simulink library "threeSurfaceThreeTether_cl"  (R2018b)
settings: Solver=VariableStepAuto  StartTime=0.0  StopTime=10.0  RelTol=1e-3
libraries: vrlib x4, turbine_ul x2, apparentWind_ul x1, eulAng2RotMat_ul x1, vectorNormalizer_ul x1, avlAerodynamics x1, sixDoFDynamics_ul x1
settings Model: Creator=mcobb  LastModifiedBy=mcobb

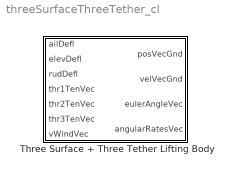
== system threeSurfaceThreeTether_cl ==
  Three Surface + Three Tether Lifting Body : Subsystem  mask{rho=1.225, vol=1, grav=9.81, thr1PosVec=[1 0 0], thr2PosVec=[1 0 0], thr3PosVec=[1 0 0], turb1Pos=0, turb2Pos=0, turbDiam=0, turbCp=0, turbCd=0, CB2CMVec=[1 0 0], m=1, inertiaMatrix=eye(3), initPos=[0 0 0], initVel=[0 0 0], initEulerAngles=[0 0 0], initAngRates=[0 0 0], hStabWingAeroCentVec=[0 0 0], hStabRotVec=[1 0 0], hStabChordVec=[0 1 0], hStabRefArea=1, hStabLiftCoeffFitParams=[1 0], hStabDragCoeffFitParams=[1 0 0], vStabWingAeroCentVec=[0 0 0], vStabRotVec=[1 0 0], vStabChordVec=[0 1 0], vStabRefArea=1, vStabLiftCoeffFitParams=[1 0], vStabDragCoeffFitParams=[1 0 0], prtWingAeroCentVec=[0 0 0], prtRotVec=[1 0 0], prtChordVec=[0 1 0], prtRefArea=1, prtLiftCoeffFitParams=[1 0], prtDragCoeffFitParams=[1 0 0], sbdWingAeroCentVec=[0 0 0], sbdRotVec=[1 0 0], sbdChordVec=[0 1 0], sbdRefArea=1, sbdLiftCoeffFitParams=[1 0], sbdDragCoeffFitParams=[1 0 0]}
      mask prompts: rho "Fuild Density"; vol "Volume"; grav "Gravity"; thr1PosVec "Tether 1"; thr2PosVec "Tether 2"; thr3PosVec "Tether 3"; turb1Pos "Turbine 1 Position Vec"; turb2Pos "Turbine 2 Position Vec"; turbDiam "Diam"; turbCp "Power Coeff"; turbCd "Drag Coeff"; CB2CMVec "CoM 2 CoB Vec"; m "Mass"; inertiaMatrix "Inertia matrix"; initPos "Initial position vec"; initVel "Initial velocity vec"; initEulerAngles "Initial euler angles"; initAngRates "Initial angular rates vec"; hStabWingAeroCentVec "Aerodynamic Center Vec"; hStabRotVec "Spanwise Rotation Vector"; hStabChordVec "Chord Direction Vec"; hStabRefArea "Ref Area"; hStabLiftCoeffFitParams "Lift Coefficient Fit Parameters"; hStabDragCoeffFitParams "Drag Coefficient Fit Parameters"; vStabWingAeroCentVec "Aerodynamic Center Vec"; vStabRotVec "Spanwise Rotation Vector"; vStabChordVec "Chord Direction Vec"; vStabRefArea "Ref Area"; vStabLiftCoeffFitParams "Lift Coefficient Fit Parameters"; vStabDragCoeffFitParams "Drag Coefficient Fit Parameters"; prtWingAeroCentVec "Aerodynamic Center Vec"; prtRotVec "Spanwise Rotation Vector"; prtChordVec "Chord Direction Vec"; prtRefArea "Ref Area"; prtLiftCoeffFitParams "Lift Coefficient Fit Parameters"; prtDragCoeffFitParams "Drag Coefficient Fit Parameters"; sbdWingAeroCentVec "Aerodynamic Center Vec"; sbdRotVec "Spanwise Rotation Vector"; sbdChordVec "Chord Direction Vec"; sbdRefArea "Ref Area"; sbdLiftCoeffFitParams "Lift Coefficient Fit Parameters"; sbdDragCoeffFitParams "Drag Coefficient Fit Parameters"
      mask DialogControl Container8 Prompt: Parameters
      mask DialogControl ParameterGroupVar Prompt: Environmental
      mask DialogControl Container3 Prompt: Tether attachment positiong vecs in body frame
      mask DialogControl Container21 Prompt: Turbines
      mask DialogControl Container4 Prompt: Cent of mass 2 cent of buoy vec
      mask DialogControl Container5 Prompt: Inertial Settings
      mask DialogControl Container11 Prompt: Horz. Stab.
      mask DialogControl Container14 Prompt: Aerodynamic Parameters
      mask DialogControl Container16 Prompt: Vert. Stab.
      mask DialogControl Container15 Prompt: Aerodynamic Parameters
      mask DialogControl Container17 Prompt: Port Wing
      mask DialogControl Container12 Prompt: Aerodynamic Parameters
      mask DialogControl Container18 Prompt: Stb. Wing
      mask DialogControl Container13 Prompt: Aerodynamic Parameters

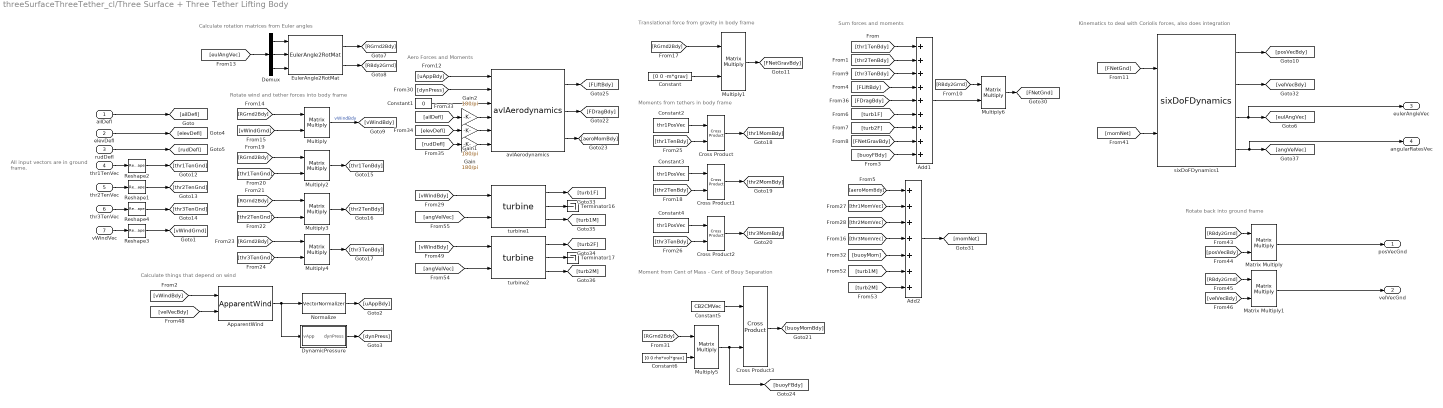
== system threeSurfaceThreeTether_cl/Three Surface + Three Tether Lifting Body ==
  note: Rotate back into ground frame
  note: Kinematics to deal with Coriolis forces, also does integration
  note: Sum forces and moments
  note: Calculate things that depend on wind
  note: Rotate wind and tether forces into body frame
  note: Calculate rotation matrices from Euler angles
  note: Moment from Cent of Mass - Cent of Bouy Separation
  note: Translational force from gravity in body frame
  note: Moments from tethers in body frame
  note: Aero Forces and Moments
  note: All input vectors are in
      | ground frame.
  ailDefl : Inport
  elevDefl : Inport  Port=2
  rudDefl : Inport  Port=3
  thr1TenVec : Inport  Port=4
  thr2TenVec : Inport  Port=5
  thr3TenVec : Inport  Port=6
  vWindVec : Inport  Port=7
  Add1 : Sum  Inputs=+++++++++
  Add2 : Sum  Inputs=+++++++
  ApparentWind : apparentWind_ul/ApparentWind  SystemSampleTime=-1
  Constant : Constant  Value=[0 0 -m*grav]
  Constant1 : Constant  Value=0
  Constant2 : Constant  Value=thr1PosVec
  Constant3 : Constant  Value=thr1PosVec
  Constant4 : Constant  Value=thr1PosVec
  Constant5 : Constant  Value=CB2CMVec
  Constant6 : Constant  Value=[0 0 rho*vol*grav]
  Cross Product{,1..3} (4 alike) : vrlib/Utilities/Cross Product
      settings: SourceProductBaseCode=VR
  Demux : Demux  Outputs=3
  DynamicPressure : Subsystem  mask{rho=rho}
      mask prompts: rho "Fluid density"
  EulerAngle2RotMat : eulAng2RotMat_ul/EulerAngle2RotMat  SystemSampleTime=-1
  Gain : Gain  Gain=180/pi
  Gain1 : Gain  Gain=180/pi
  Gain2 : Gain  Gain=180/pi
  Matrix Multiply : Product  Multiplication=Matrix(*)
  Matrix Multiply1 : Product  Multiplication=Matrix(*)
  Multiply{,1..6} (7 alike) : Product  Multiplication=Matrix(*)
  "Normalize " : vectorNormalizer_ul/VectorNormalizer   SystemSampleTime=-1
  Reshape{1..4} (4 alike) : Reshape  OutputDimensionality=Column vector (2-D)
  Terminator16 : Terminator
  Terminator17 : Terminator
  avlAerodynamics : avlAerodynamics/avlAerodynamics  CLTable=CLtotTbl  CDTable=CLtotTbl  CMxTable=CLtotTbl  CMyTable=CLtotTbl  CMzTable=CLtotTbl  SRef=0  BRef=0  CRef=0
  sixDoFDynamics1 : sixDoFDynamics_ul/sixDoFDynamics  m=1  initPos=0  initVel=0  J=eye(3)  initEulAngs=0  initAngVel=0
  turbine1 : turbine_ul/turbine  diam=turbDiam  Cp=turbCp  Cd=turbCd  rho=rho  rTurb=turb1Pos
  turbine2 : turbine_ul/turbine  diam=turbDiam  Cp=turbCp  Cd=turbCd  rho=rho  rTurb=turb2Pos
  posVecGnd : Outport
  velVecGnd : Outport  Port=2
  eulerAngleVec : Outport  Port=3
  angularRatesVec : Outport  Port=4
  wires:
  ailDefl/1 -> [ailDefl]
  vWindVec/1 -> Reshape3/1
  [vWindGrnd] -> Multiply/2
  ApparentWind/1 -> "Normalize "/1, DynamicPressure/1(vApp)
  "Normalize "/1 -> [uAppBdy]
  DynamicPressure/1(dynPress) -> [dynPress]
  elevDefl/1 -> [elevDefl]
  rudDefl/1 -> [rudDefl]
  [eulAngVec] -> Demux/1
  Demux/2 -> EulerAngle2RotMat/2
  Demux/1 -> EulerAngle2RotMat/1
  Demux/3 -> EulerAngle2RotMat/3
  EulerAngle2RotMat/1 -> [RGrnd2Bdy]
  EulerAngle2RotMat/2 -> [RBdy2Grnd]
  [RGrnd2Bdy] -> Multiply/1
  Multiply/1 -> [vWindBdy]  "vWindBdy"
  [vWindBdy] -> ApparentWind/1
  [velVecBdy] -> ApparentWind/2
  [RGrnd2Bdy] -> Multiply1/1
  Multiply1/1 -> [FNetGravBdy]
  thr1TenVec/1 -> Reshape2/1
  thr2TenVec/1 -> Reshape1/1
  thr3TenVec/1 -> Reshape4/1
  Multiply2/1 -> [thr1TenBdy]
  [RGrnd2Bdy] -> Multiply2/1
  [thr1TenGnd] -> Multiply2/2
  [thr2TenGnd] -> Multiply3/2
  [RGrnd2Bdy] -> Multiply3/1
  Multiply3/1 -> [thr2TenBdy]
  Multiply4/1 -> [thr3TenBdy]
  [RGrnd2Bdy] -> Multiply4/1
  [thr3TenGnd] -> Multiply4/2
  [thr1TenBdy] -> Cross Product/2
  Constant2/1 -> Cross Product/1
  Cross Product/1 -> [thr1MomBdy]
  Cross Product1/1 -> [thr2MomBdy]
  Constant3/1 -> Cross Product1/1
  [thr2TenBdy] -> Cross Product1/2
  [thr3TenBdy] -> Cross Product2/2
  Constant4/1 -> Cross Product2/1
  Cross Product2/1 -> [thr3MomBdy]
  Constant6/1 -> Multiply5/2
  Multiply5/1 -> [buoyFBdy], Cross Product3/2
  [RGrnd2Bdy] -> Multiply5/1
  Cross Product3/1 -> [buoyMomBdy]
  Constant5/1 -> Cross Product3/1
  Add1/1 -> Multiply6/2
  [aeroMomBdy] -> Add2/1
  [thr2MomVec] -> Add2/3
  [thr1MomVec] -> Add2/2
  Add2/1 -> [momNet]
  [momNet] -> sixDoFDynamics1/2
  [FNetGnd] -> sixDoFDynamics1/1
  sixDoFDynamics1/3 -> [eulAngVec], eulerAngleVec/1
  sixDoFDynamics1/1 -> [posVecBdy]
  sixDoFDynamics1/2 -> [velVecBdy]
  sixDoFDynamics1/4 -> [angVelVec], angularRatesVec/1
  [RBdy2Grnd] -> Matrix Multiply/1
  Matrix Multiply/1 -> posVecGnd/1
  [posVecBdy] -> Matrix Multiply/2
  [velVecBdy] -> Matrix Multiply1/2
  [RBdy2Grnd] -> Matrix Multiply1/1
  Matrix Multiply1/1 -> velVecGnd/1
  Reshape2/1 -> [thr1TenGnd]
  Reshape1/1 -> [thr2TenGnd]
  Reshape4/1 -> [thr3TenGnd]
  Reshape3/1 -> [vWindGrnd]
  [vWindBdy] -> turbine1/1
  [vWindBdy] -> turbine2/1
  turbine1/1 -> [turb1F]
  turbine2/1 -> [turb2F]
  turbine1/2 -> Terminator16/1
  turbine2/2 -> Terminator17/1
  turbine1/3 -> [turb1M]
  turbine2/3 -> [turb2M]
  [angVelVec] -> turbine2/2
  [angVelVec] -> turbine1/2
  [thr1TenBdy] -> Add1/1
  [thr2TenBdy] -> Add1/2
  [thr3TenBdy] -> Add1/3
  Constant/1 -> Multiply1/2
  [turb2M] -> Add2/7
  [turb1M] -> Add2/6
  [buoyMom] -> Add2/5
  [thr3MomVec] -> Add2/4
  Multiply6/1 -> [FNetGnd]
  [RBdy2Grnd] -> Multiply6/1
  avlAerodynamics/3 -> [aeroMomBdy]
  avlAerodynamics/2 -> [FDragBdy]
  avlAerodynamics/1 -> [FLiftBdy]
  [uAppBdy] -> avlAerodynamics/1
  [dynPress] -> avlAerodynamics/2
  Constant1/1 -> avlAerodynamics/3
  [rudDefl] -> Gain/1
  Gain/1 -> avlAerodynamics/6
  [elevDefl] -> Gain1/1
  Gain1/1 -> avlAerodynamics/5
  [ailDefl] -> Gain2/1
  Gain2/1 -> avlAerodynamics/4
  [buoyFBdy] -> Add1/9
  [FNetGravBdy] -> Add1/8
  [turb2F] -> Add1/7
  [turb1F] -> Add1/6
  [FLiftBdy] -> Add1/4
  [FDragBdy] -> Add1/5

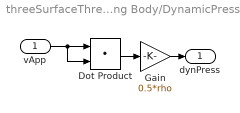
== system threeSurfaceThreeTether_cl/Three Surface + Three Tether Lifting Body/DynamicPressure ==
  vApp : Inport
  Dot Product : DotProduct  InputSameDT=on  OutDataTypeStr=Inherit: Inherit via internal rule
  Gain : Gain  Gain=0.5*rho
  dynPress : Outport
  wires:
  Dot Product/1 -> Gain/1
  vApp/1 -> Dot Product/1, Dot Product/2
  Gain/1 -> dynPress/1
